simulink library "Storage_Type_2"  (R2016b)
settings: Solver=ode45  StartTime=0.0  StopTime=10.0  RelTol=1e-3  EnableMultiTasking=on
libraries: carnot x10
settings Model: Creator=lena.frank  LastModifiedBy=drhf
settings DataIOCC: LimitDataPoints=on  SaveFormat=Array  SignalLoggingSaveFormat=ModelDataLogs
settings OptimizationCC: ExpressionDepthLimit=2147483647  LifeSpan=inf
settings DebuggingCC: UnderspecifiedInitializationDetection=Classic  MergeDetectMultiDrivingBlocksExec=none  SolverPrmCheckMsg=warning  FcnCallInpInsideContextMsg=warning  StateNameClashWarn=warning  SFUnexpectedBacktrackingDiag=warning  SFNoUnconditionalDefaultTransitionDiag=warning  SFExecutionAtInitializationDiag=none
settings HardwareCC: ProdBitPerPointer=32  ProdBitPerSizeT=32  ProdBitPerPtrDiffT=32  ProdLargestAtomicFloat=None  ProdIntDivRoundTo=Undefined  ProdEndianess=Unspecified  ProdWordSize=32  ProdHWDeviceType=32-bit Generic
settings ModelReferenceCC: PropagateSignalLabelsOutOfModel=off
settings GRTTargetCC: TargetLangStandard=C89/C90 (ANSI)  GeneratePreprocessorConditionals=Disable all  CombineOutputUpdateFcns=off  GRTInterface=on
settings ConfigComp: CovMetricSettings=dw  CovHtmlReporting=on  CovSaveCumulativeToWorkspaceVar=on  CovSaveSingleToWorkspaceVar=on  CovExternalEMLEnable=off

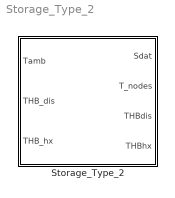
== system Storage_Type_2 ==
  Storage_Type_2 : Subsystem  mask(Multiport Storage){uloss=1, ubot=1, utop=1, cond=1, volume=0.3, dia=0.5, pos=standing cylinder, h_in_chg=0.5, h_out_chg=0.1, ua0=80, uam=0.2, uat=0.5, dplin_chg=100, dpqua_chg=100, h_in=0, h_out=1, pipedia=0.03, t0=60, nodes=10, mpoints=10}
      mask prompts: uloss "heat transfer coefficient to ambient [W/m²K]"; ubot "heat transfer coefficient to ambient bottom [W/m²K]"; utop "heat transfer coefficient to ambient top [W/m²K]"; cond "effective thermal conductivity [W/mK]"; volume "Volume [m³]"; dia "diameter [m]"; pos "Position"; h_in_chg "relative height of inlet, range = 0 (bottom) to 1 (top)"; h_out_chg "relative height of outlet, range = 0 (bottom) to 1 (top)"; ua0 "uac - constant heat transfer coefficient [W/K]"; uam "uam - massflow dependent heat transfer [W*s/(K*kg)]"; uat "uat - temperature difference dependent heat transfer [W/K²]"; dplin_chg "pressure drop linear in mdot [Pa*s/kg]"; dpqua_chg "pressure drop quadratic in mdot [Pa*s²/kg²]"; h_in "relative height of inlet , range = 0 (bottom) to 1 (top)"; h_out "relative height of outlet, range = 0 (bottom) to 1 (top)"; pipedia "Diameter of pipe in m"; t0 "Initial temperature (vector or scalar) in °C"; nodes "Number of nodes"; mpoints "Number of measurement points"
      mask help:
      | The volmue of the cylindrical storage is divided in a number "nodes" of horizontal slices (1xN-node model). For each node the energy balance equation is solved.
      | Parameters from underlying sub-masks are promoted by top mask.
      mask init:
      | [standing, dh, height, mpts, tini] ...
      |     = CarnotCallbacks_StorageTypeN(pos, volume, dia, nodes, mpoints, t0);
      mask Help: web(fullfile(path_carnot('help'),'Storage_Type_N.html'),'-helpbrowser')
      mask TypeOptions uloss: sfun_storageTnodes/uloss
      mask TypeOptions ubot: sfun_storageTnodes/ubot
      mask TypeOptions utop: sfun_storageTnodes/utop
      mask TypeOptions cond: sfun_storageTnodes/cond
      mask TypeOptions volume: sfun_storageTnodes/volume | CreateSdat/volume
      mask TypeOptions dia: sfun_storageTnodes/dia
      mask TypeOptions pos: lying cylinder | standing cylinder
      mask TypeOptions h_in_chg: HX_data_fit/h_in
      mask TypeOptions h_out_chg: HX_data_fit/h_out
      mask TypeOptions ua0: HX_data_fit/ua0
      mask TypeOptions uam: HX_data_fit/uam
      mask TypeOptions uat: HX_data_fit/uat
      mask TypeOptions dplin_chg: HX_data_fit/dplin
      mask TypeOptions dpqua_chg: HX_data_fit/dpqua
      mask TypeOptions h_in: pipe/h_in
      mask TypeOptions h_out: pipe/h_out
      mask TypeOptions pipedia: pipe/dia
      mask TypeOptions nodes: sfun_storageTnodes/nodes | select_T/InputPortWidth | pipe/nodes
      mask Display: plot(10,20,80,100,[36,36,40,50,54,54,50,40,36],[90,50,45,45,50,90,93,93,90],[36,51,44,51,36],[50,50,55,60,60])

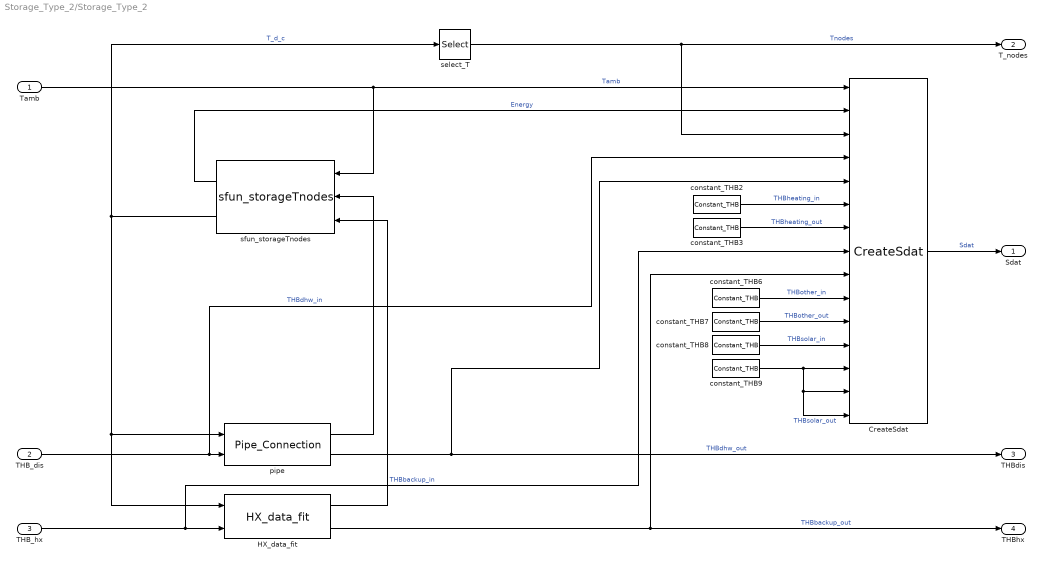
== system Storage_Type_2/Storage_Type_2 ==
  Tamb : Inport
  THB_dis : Inport  Port=2
  THB_hx : Inport  Port=3
  CreateSdat : carnot/Basic/Thermal_Models/CreateSdat  volume=volume  stgtype=1
  HX_data_fit : carnot/Storage/Thermal/Storage_Ports/HX_data_fit  h_in=h_in_chg  h_out=h_out_chg  hgt=height  dia=dia  ua0=ua0  uam=uam  uat=uat  dplin=dplin_chg  dpqua=dpqua_chg  nodes=nodes
  constant_THB{2..3,6..9} (6 alike) : carnot/Source/Simple/Constant_THB  t=20  mdot=0  p=1e5  mID=No Pressure Drop  fluid=Water  mix=0  mix2=0  mix3=0  dia=0.02  hgt=0
  pipe : carnot/Storage/Thermal/Storage_Ports/Pipe_Connection  h_in=h_in  h_out=h_out  hgt=height  dia=pipedia  nodes=nodes
  select_T : Selector  InputPortWidth=nodes  IndexOptions=Index vector (dialog)  Indices=mpts  OutputSizes=1
  sfun_storageTnodes : carnot/Basic/Thermal_Models/sfun_storageTnodes  uloss=uloss  ubot=ubot  utop=utop  cond=cond  volume=volume  dia=dia  standing=standing cylinder  tini=tini  nodes=nodes  nconnect=2  elimthermocline=2  condinvtc=1e5
  Sdat : Outport
  T_nodes : Outport  Port=2
  THBdis : Outport  Port=3
  THBhx : Outport  Port=4
  wires:
  THB_hx/1 -> CreateSdat/8, HX_data_fit/2  "THBbackup_in"
  THB_dis/1 -> CreateSdat/4, pipe/2  "THBdhw_in"
  select_T/1 -> CreateSdat/3, T_nodes/1  "Tnodes"
  Tamb/1 -> CreateSdat/1, sfun_storageTnodes/1  "Tamb"
  pipe/2 -> CreateSdat/5, THBdis/1  "THBdhw_out"
  pipe/1 -> sfun_storageTnodes/2
  sfun_storageTnodes/1 -> CreateSdat/2  "Energy"
  sfun_storageTnodes/2 -> select_T/1, pipe/1, HX_data_fit/1  "T_d_c"
  CreateSdat/1 -> Sdat/1  "Sdat"
  constant_THB9/1 -> CreateSdat/13, CreateSdat/14, CreateSdat/15  "THBsolar_out"
  constant_THB8/1 -> CreateSdat/12  "THBsolar_in"
  constant_THB7/1 -> CreateSdat/11  "THBother_out"
  constant_THB6/1 -> CreateSdat/10  "THBother_in"
  constant_THB2/1 -> CreateSdat/6  "THBheating_in"
  constant_THB3/1 -> CreateSdat/7  "THBheating_out"
  HX_data_fit/2 -> CreateSdat/9, THBhx/1  "THBbackup_out"
  HX_data_fit/1 -> sfun_storageTnodes/3
